simulink model "fullmod"  (R2014b)
settings: Solver=ode45  StartTime=0.0  StopTime=10  MaxStep=0.001  MinStep=0.0001  RelTol=1e-3
values from neighbouring files (symbols this model uses):
  ip = 16    [lab10.m]    (also in work.mat; work2.mat; work3.mat; work4.mat)
  Jsum = Jd+Jp+(Jm/(ip^2))    (= 0.0126621875)    [lab10.m]    (also in work.mat; work2.mat; work3.mat; work4.mat)
  Kd = 1/R    (= 1.33333333333)    [lab10.m]    (also in work.mat; work2.mat; work3.mat; work4.mat)
  Ke = Un/Angular_velocity    (= 0.716195569137)    [lab10.m]    (also in work.mat; work2.mat; work3.mat; work4.mat)
  Km = Mn/In    (= 0.458333333333)    [lab10.m]    (also in work.mat; work2.mat; work3.mat; work4.mat)
  Ky = Un/Um    (= 7.5)    [lab10.m]    (also in work.mat; work2.mat; work3.mat; work4.mat)
  Tja = 5/1000    (= 0.005)    [lab10.m]    (also in work.mat; work2.mat; work3.mat; work4.mat)
  Ty = 6/1000    (= 0.006)    [lab10.m]    (also in work.mat; work2.mat; work3.mat; work4.mat)
settings Model: Creator=Игорь  LastModifiedBy=Игорь

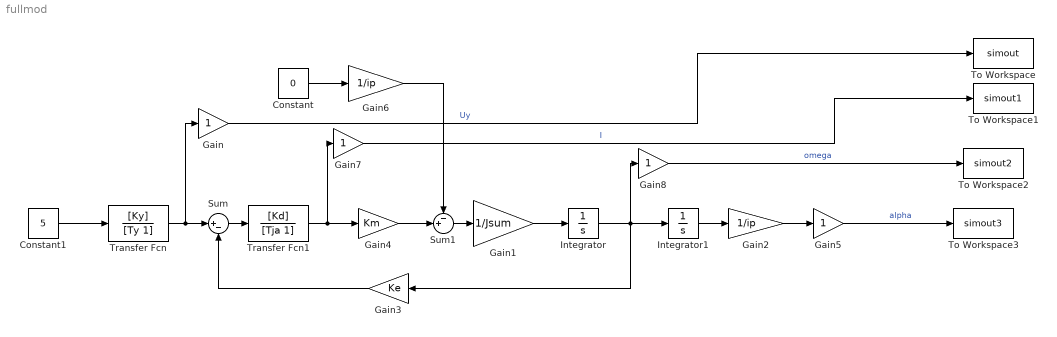
== system fullmod ==
  Constant : Constant  Value=0
  Constant1 : Constant  Value=5
  Gain{,5,7..8} (4 alike) : Gain
  Gain1 : Gain  Gain=1/Jsum
  Gain2 : Gain  Gain=1/ip
  Gain3 : Gain  Gain=Ke
  Gain4 : Gain  Gain=Km
  Gain6 : Gain  Gain=1/ip
  Integrator : Integrator
  Integrator1 : Integrator
  Sum : Sum  Inputs=|+-
  Sum1 : Sum  Inputs=-+|
  To Workspace : ToWorkspace  VariableName=simout  SaveFormat=Timeseries  SampleTime=-1
  To Workspace1 : ToWorkspace  VariableName=simout1  SaveFormat=Timeseries  SampleTime=-1
  To Workspace2 : ToWorkspace  VariableName=simout2  SaveFormat=Timeseries  SampleTime=-1
  To Workspace3 : ToWorkspace  VariableName=simout3  SaveFormat=Timeseries  SampleTime=-1
  Transfer Fcn : TransferFcn  Numerator=[Ky]  Denominator=[Ty 1]
  Transfer Fcn1 : TransferFcn  Numerator=[Kd]  Denominator=[Tja 1]
  wires:
  Transfer Fcn/1 -> Gain/1, Sum/1
  Sum/1 -> Transfer Fcn1/1
  Gain3/1 -> Sum/2
  Transfer Fcn1/1 -> Gain7/1, Gain4/1
  Gain4/1 -> Sum1/2
  Sum1/1 -> Gain1/1
  Gain1/1 -> Integrator/1
  Integrator/1 -> Gain3/1, Gain8/1, Integrator1/1
  Integrator1/1 -> Gain2/1
  Constant/1 -> Gain6/1
  Gain6/1 -> Sum1/1
  Gain2/1 -> Gain5/1
  Constant1/1 -> Transfer Fcn/1
  Gain/1 -> To Workspace/1  "Uy"
  Gain7/1 -> To Workspace1/1  "I"
  Gain8/1 -> To Workspace2/1  "omega"
  Gain5/1 -> To Workspace3/1  "alpha"
